simulink model "Quadruple_Tank_Simulation"  (R2021b)
settings: Solver=VariableStepAuto  StartTime=0.0  StopTime=200  MaxStep=0.1  RelTol=1e-3
values from neighbouring files (symbols this model uses):
  a1 = 0.17795237427    [Dados_Tanques.mat]    (also in double_tank_simu.m)
  A1 = 15.5179165474    [Dados_Tanques.mat]    (also in double_tank_simu.m)
  a2 = 0.17795237427    [Dados_Tanques.mat]    (also in double_tank_simu.m)
  A2 = 15.5179165474    [Dados_Tanques.mat]    (also in double_tank_simu.m)
  g = 981    [Dados_Tanques.mat]    (also in double_tank_simu.m)
  x1eq = 15    [Dados_Tanques.mat]    (also in double_tank_simu.m = (1/(2*g))*((km*ueq)/a1)^2)
  x2eq = 15    [Dados_Tanques.mat]    (also in double_tank_simu.m)
undefined symbols (not defined in the file or in its folder): a3, A3, a4, A4, ans, k1, k2, q1, q2, u1eq, u2eq, x3eq, x4eq
libraries: instrumentlib x2
settings Model: Creator=mathe  LastModifiedBy=mathe

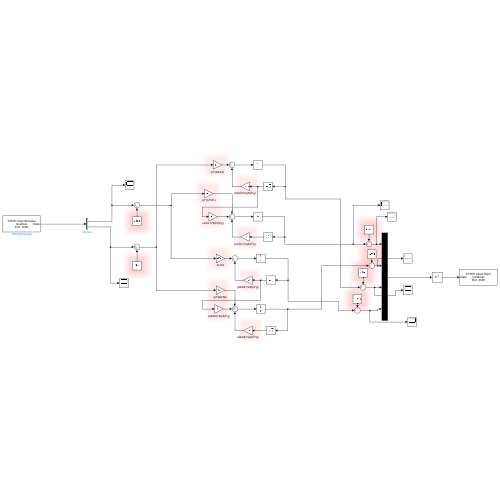
[thumbnail: Simulink's stored preview of the top-level diagram]
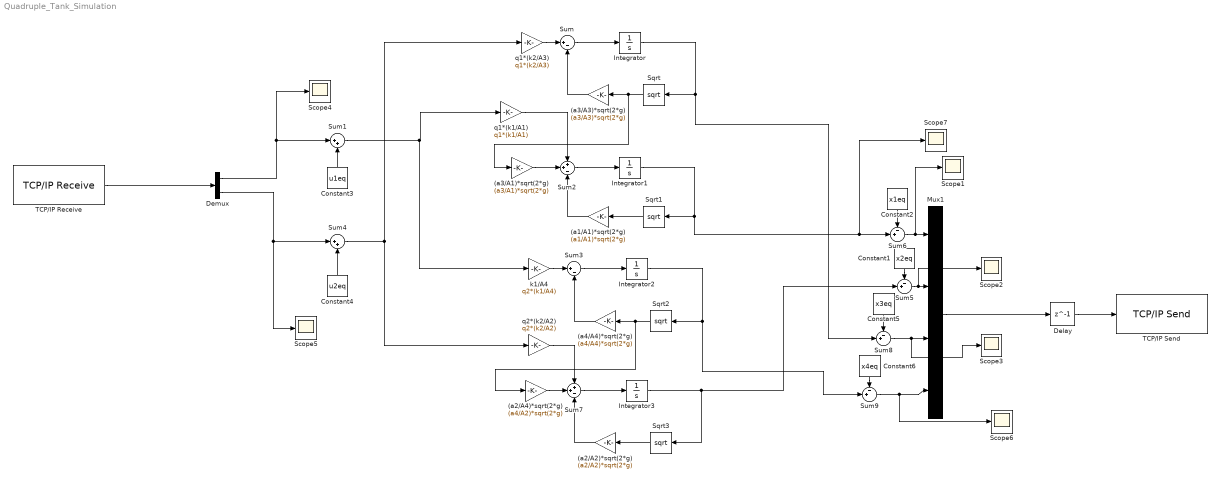
== system Quadruple_Tank_Simulation ==
  (a1/A1)*sqrt(2*g) : Gain  Gain=(a1/A1)*sqrt(2*g)
  (a2/A2)*sqrt(2*g) : Gain  Gain=(a2/A2)*sqrt(2*g)
  (a2/A4)*sqrt(2*g) : Gain  Gain=(a4/A2)*sqrt(2*g)
  (a3/A1)*sqrt(2*g) : Gain  Gain=(a3/A1)*sqrt(2*g)
  (a3/A3)*sqrt(2*g) : Gain  Gain=(a3/A3)*sqrt(2*g)
  (a4/A4)*sqrt(2*g) : Gain  Gain=(a4/A4)*sqrt(2*g)
  Constant1 : Constant  Value=x2eq
  Constant2 : Constant  Value=x1eq
  Constant3 : Constant  Value=u1eq
  Constant4 : Constant  Value=u2eq
  Constant5 : Constant  Value=x3eq
  Constant6 : Constant  Value=x4eq
  Delay : Delay  DelayLength=1  InitialCondition=0
  Demux : Demux  Outputs=2
  Integrator : Integrator  InitialCondition=ans(3)
  Integrator1 : Integrator  InitialCondition=ans(1)
  Integrator2 : Integrator  InitialCondition=ans(4)
  Integrator3 : Integrator  InitialCondition=ans(2)
  Mux1 : Mux
  Scope{1..7} (7 alike) : Scope
  Sqrt{,1..3} (4 alike) : Sqrt  SaturateOnIntegerOverflow=on
  Sum : Sum  Inputs=|+-
  Sum1 : Sum  Inputs=|++
  Sum2 : Sum  Inputs=++-
  Sum3 : Sum  Inputs=|+-
  Sum4 : Sum  Inputs=|++
  Sum{5..6,8..9} (4 alike) : Sum  Inputs=-+|
  Sum7 : Sum  Inputs=++-
  TCP/IP Receive : instrumentlib/TCP//IP Receive  Priority=2  Host=localhost  Port=3000  DataSize=[ 2, 1 ]  DataType=double  ASCIIFormatting=%f  Terminator=LF  CustomTerminator=10  ByteOrder=big-endian  EnableBlockingMode=on  Timeout=200  SampleTime=0.1  SimulateUsing=Interpreted execution
  TCP/IP Send : instrumentlib/TCP//IP Send  Priority=1  Host=localhost  Port=3000  ByteOrder=big-endian  EnableBlockingMode=on  Timeout=500  TransferDelay=off  SimulateUsing=Interpreted execution
  k1/A4 : Gain  Gain=q2*(k1/A4)
  q1*(k1/A1) : Gain  Gain=q1*(k1/A1)
  q1*(k2/A3) : Gain  Gain=q1*(k2/A3)
  q2*(k2/A2) : Gain  Gain=q2*(k2/A2)
  wires:
  Sum4/1 -> q2*(k2/A2)/1, q1*(k2/A3)/1
  Sum1/1 -> k1/A4/1, q1*(k1/A1)/1
  q2*(k2/A2)/1 -> Sum7/1
  Sqrt3/1 -> (a2/A2)*sqrt(2*g)/1
  Integrator/1 -> Sum8/2, Sqrt/1
  Integrator2/1 -> Sum9/2, Sqrt2/1
  Sum2/1 -> Integrator1/1
  (a3/A3)*sqrt(2*g)/1 -> Sum/2
  Sum3/1 -> Integrator2/1
  Sum/1 -> Integrator/1
  Integrator3/1 -> Sum5/2, Sqrt3/1
  Sqrt2/1 -> (a2/A4)*sqrt(2*g)/1, (a4/A4)*sqrt(2*g)/1
  Sqrt/1 -> (a3/A1)*sqrt(2*g)/1, (a3/A3)*sqrt(2*g)/1
  q1*(k2/A3)/1 -> Sum/1
  Sqrt1/1 -> (a1/A1)*sqrt(2*g)/1
  (a2/A4)*sqrt(2*g)/1 -> Sum7/2
  (a2/A2)*sqrt(2*g)/1 -> Sum7/3
  Sum7/1 -> Integrator3/1
  k1/A4/1 -> Sum3/1
  (a4/A4)*sqrt(2*g)/1 -> Sum3/2
  (a1/A1)*sqrt(2*g)/1 -> Sum2/3
  Integrator1/1 -> Sqrt1/1, Scope7/1, Sum6/2
  (a3/A1)*sqrt(2*g)/1 -> Sum2/2
  q1*(k1/A1)/1 -> Sum2/1
  TCP/IP Receive/1 -> Demux/1
  Constant4/1 -> Sum4/2
  Demux/1 -> Scope4/1, Sum1/1
  Constant3/1 -> Sum1/2
  Demux/2 -> Scope5/1, Sum4/1
  Sum6/1 -> Scope1/1, Mux1/1
  Constant2/1 -> Sum6/1
  Sum5/1 -> Scope2/1, Mux1/2
  Constant1/1 -> Sum5/1
  Sum8/1 -> Scope3/1, Mux1/3
  Constant5/1 -> Sum8/1
  Sum9/1 -> Scope6/1, Mux1/4
  Constant6/1 -> Sum9/1
  Mux1/1 -> Delay/1
  Delay/1 -> TCP/IP Send/1
